simulink model "simulink_panda"  (R2019b)
settings: Solver=ode1  StartTime=0.0  StopTime=tf  FixedStep=0.01  RelTol=1e-3
values from neighbouring files (symbols this model uses):
  qi = [pi/2 ; 0 ; 0 ;-pi/2 ; 0 ;pi/2 ; pi/6]    [sim_panda.m]
settings Model: Creator=mahdie  LastModifiedBy=mahdie

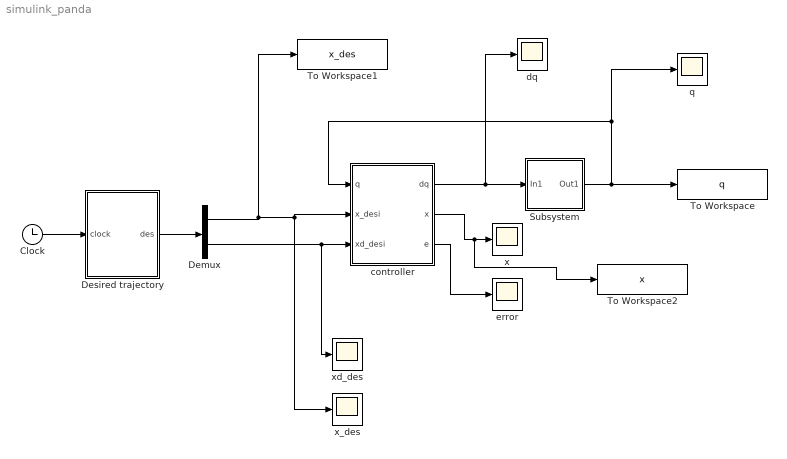
== system simulink_panda ==
  Clock : Clock
      settings: Decimation=6
  Demux : Demux  Outputs=2
  Desired trajectory : MATLAB Function  TreatAsAtomicUnit=on
  Subsystem : Subsystem
  To Workspace : ToWorkspace  VariableName=q  SampleTime=-1
  To Workspace1 : ToWorkspace  VariableName=x_des  SampleTime=-1
  To Workspace2 : ToWorkspace  VariableName=x  SampleTime=-1
  "controller " : MATLAB Function  TreatAsAtomicUnit=on
  dq : Scope
  error : Scope
  q : Scope
  x : Scope
  "x_des " : Scope
  xd_des : Scope
  wires:
  Subsystem/1(Out1) -> To Workspace/1, "controller "/1(q), q/1
  Demux/2 -> xd_des/1, "controller "/3(xd_desi)
  "controller "/1(dq) -> dq/1, Subsystem/1(In1)
  Desired trajectory/1(des) -> Demux/1
  Demux/1 -> To Workspace1/1, "x_des "/1, "controller "/2(x_desi)
  Clock/1 -> Desired trajectory/1(clock)
  "controller "/2(x) -> To Workspace2/1, x/1
  "controller "/3(e) -> error/1

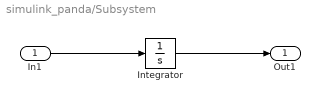
== system simulink_panda/Subsystem ==
  In1 : Inport
  Integrator : Integrator  InitialCondition=qi
  Out1 : Outport
  wires:
  In1/1 -> Integrator/1
  Integrator/1 -> Out1/1

== matlab function simulink_panda/controller  ==
  data: q input; dq output; x_desi input; xd_desi input; x output; e output
function [dq,x,e] = fcn(q,x_desi,xd_desi)
teta1=q(1);
teta2=q(2);
teta3=q(3);
teta4=q(4);
teta5=q(5);
teta6=q(6);
teta7=q(7);  

%% jacobian
A=cell(7);
T0=cell(7);
R0=cell(7);
P0=cell(7);
Z=cell(7);

teta=[teta1 teta2 teta3 teta4 teta5 teta6 teta7];
alpha=[pi/2 -pi/2 pi/2 -pi/2 pi/2 pi/2 0];
a=[0 0 0.0825 -0.0825 0 0.088 0];
d=[0.333 0 0.316 0 0.384 0 0.1070];

for i=1:7
    A{i-1+1,i}=[cos(teta(i)) -sin(teta(i))*cos(alpha(i)) sin(teta(i))*sin(alpha(i)) a(i)*cos(teta(i));
    sin(teta(i)) cos(teta(i))*cos(alpha(i)) -cos(teta(i))*sin(alpha(i)) a(i)*sin(teta(i));
    0 sin(alpha(i)) cos(alpha(i)) d(i);
    0 0 0 1];
end

T0{1}=A{1-1+1,1};
for i=2:7
    T0{i}=T0{i-1}*A{i-1+1,i};
end
for i=1:7
    R0{i}=T0{i}(1:3,1:3);
    P0{i}=T0{i}(1:3,4);
end
Z{0+1}=[0 0 1]';
for i=1:7
    Z{i+1}=R0{i}*[0 0 1]';
end
j=[cross(Z{0+1},P0{7}) cross(Z{1+1},P0{7}-P0{1}) cross(Z{1+2},P0{7}-P0{2}) cross(Z{1+3},P0{7}-P0{3}) cross(Z{1+4},P0{7}-P0{4}) cross(Z{1+5},P0{7}-P0{5}) cross(Z{1+6},P0{7}-P0{6});
    Z{0+1} Z{1+1} Z{2+1} Z{3+1} Z{4+1} Z{5+1} Z{6+1}];

%analyitic
rzyz=rotm2eul(T0{7}(1:3,1:3),'xyz');
Tzyz=[1 0 sin(rzyz(2));0 cos(rzyz(1)) -cos(rzyz(2))*sin(rzyz(1));0 sin(rzyz(1)) cos(rzyz(2))*cos(rzyz(1))];
v=[eye(3) zeros(3);zeros(3) Tzyz];
j=inv(v)*j;

r=rotm2eul(T0{7}(1:3,1:3),'xyz');
if r(1)<-3.14
    r(1)=-r(1);
end
x=[T0{7}(1:3,4);r(1);r(2);r(3)];

detj= det(j*j.');
if detj<0.5
 k=(1-(detj/0.5)^2)*0.2;
else
    k=0;
end

jstar=j.'*inv((j*j.'+k*eye(6)));
landa=[200 0 0 0 0 0;0 200 0 0 0 0;0 0 200 0 0 0;0 0 0 50 0 0;0 0 0 0 100 0;0 0 0 0 0 100];
dq=jstar*(xd_desi+landa*(x_desi-x));
e=(x_desi-x);

== matlab function simulink_panda/Desired trajectory ==
  data: des output; clock input
function des = fcn(clock)
t=clock;

pinitial=[0 0.5545 0.6245 3.1416 0 -1.0472].';
pf=[0.2689 0.2689 0.0359 3.1416 0 -1.0472].';

%% trajectory
l=norm(pf-pinitial);
vmax=0.18;
T=7;
ts=T-l/vmax;
amax=vmax/ts;

    if t<=ts
        sigma=amax*t^2/2;
        sigmadot=amax*t;
    elseif (ts<t)&&(t<T-ts)
        sigma=vmax*t-vmax^2/(2*amax);
        sigmadot=vmax;
    else
        sigma=-amax*((t-T)^2)/2+vmax*T-vmax^2/amax;
        sigmadot=-amax*(t-T);
    end

ps= pinitial+(sigma/l).*(pf-pinitial);
des=[ps;(sigmadot/l).*(pf-pinitial)];
